simulink model "rtwdemo_autosar_client"  (Simulink 7.6)
settings: Solver=FixedStepDiscrete  SolverMode=SingleTasking  StartTime=0.0  StopTime=10.0  FixedStep=0.1  RelTol=1e-3
libraries: rtwdemo_autosar_csinterface x2, rtwlib x1
Description:
  | File Packaging for Models (Code and Data)
settings Model: Creator=The MathWorks Inc.  ExtModeAutoUpdateStatusClock=off
settings MATStruct: SampleTime=0.1  Offset=0  Priority=[20.0]
settings DataIOCC: LimitDataPoints=off  SaveFormat=StructureWithTime  SaveOutput=off  SaveTime=off  SignalLoggingName=logsOut
settings OptimizationCC: InlineParams=on  InlineInvariantSignals=on  StateBitsets=on  DataBitsets=on  UseTempVars=on  ZeroExternalMemoryAtStartup=off  ZeroInternalMemoryAtStartup=off  EfficientFloat2IntCast=on  EfficientMapNaN2IntZero=off  OptimizeModelRefInitCode=on  LifeSpan=floor((10.0)/86400)+1
settings DebuggingCC: CheckExecutionContextPreStartOutputMsg=on  CheckExecutionContextRuntimeOutputMsg=on  SolverPrmCheckMsg=none  StrictBusMsg=ErrorOnBusTreatedAsVector
settings HardwareCC: ProdIntDivRoundTo=Zero  ProdEndianess=LittleEndian  ProdHWDeviceType=Generic->32-bit Embedded Processor  TargetHWDeviceType=Generic->32-bit Embedded Processor
settings ModelReferenceCC: UpdateModelReferenceTargets=IfOutOfDate  CheckModelReferenceTargetMessage=none
settings RTWCC: SystemTargetFile=autosar.tlc  TLCOptions=-p0 -aWarnNonSaturatedBlocks=0  GenCodeOnly=on  TemplateMakefile=ert_default_tmf  Description=AUTOSAR  GenerateReport=on  RTWVerbose=off  ProcessScript=autosar_make_rtw_hook  IncludeHyperlinkInReport=on  LaunchReport=on  GenerateCodeInfo=on
settings CodeAppCC: ForceParamTrailComments=on  IgnoreCustomStorageClasses=off  MaxIdLength=128
settings STFCustomTargetCC: ParMdlRefBuildCompliant=on  CompOptLevelCompliant=on  IncludeMdlTerminateFcn=off  CombineOutputUpdateFcns=on  SuppressErrorStatus=on  ERTFirstTimeCompliant=on  ERTCustomFileBanners=on  SupportNonFinite=off  SupportComplex=off  SupportContinuousTime=off  SupportNonInlinedSFcns=off  AutosarCompliant=on  SystemTargetFile=autosar.tlc
settings ERTTargetCC: MultiwordLength=2048  IncludeMdlTerminateFcn=off  SuppressErrorStatus=on  SupportNonFinite=off  SupportComplex=off  ModelStepFunctionPrototypeControlCompliant=off  CPPClassGenCompliant=off  AutosarCompliant=on  ExtModeMexFile=noextcomm  InlinedParameterPlacement=NonHierarchical  ERTCustomFileTemplate=example_file_process.tlc  ERTFilePackagingFormat=CompactWithDataFile  ConvertIfToSwitch=off
settings CustomProperty: DataType=RTWOptions_EnumType__toolbox_rtw_targets_AUTOSAR_AUTOSAR_autosar_1_1AutosarSchemaVersion  Value=3.1
settings EnumStrPairs: String=2.0

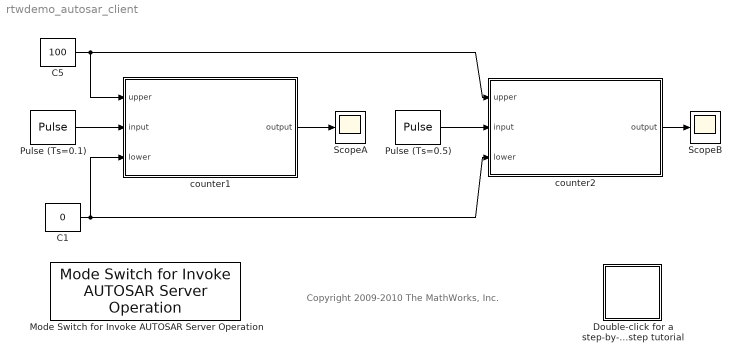
== system rtwdemo_autosar_client ==
  note: Copyright 2009-2010 The MathWorks, Inc.
  C1 : Constant  Value=0
  C5 : Constant  Value=100
  Double-click for a step-by-step tutorial : Subsystem
      settings: OpenFcn=showdemo('rtwdemo_autosar_clientserver_script');
      mask Type: Info
      mask Display: image(imread('targets_demo_info.bmp','bmp'),'center')
  Mode Switch for Invoke AUTOSAR Server Operation : rtwlib/AUTOSAR/Mode Switch for Invoke AUTOSAR Server Operation  SystemSampleTime=-1  mode=code generation  ShowInLibBrowser=on
  Pulse (Ts=0.1) : DiscretePulseGenerator  SampleTime=0.1  VectorParams1D=off
  Pulse (Ts=0.5) : DiscretePulseGenerator  SampleTime=0.5
  ScopeA : Scope
      settings: TimeRange=10  YMin=0  YMax=100
  ScopeB : Scope
      settings: TimeRange=10  YMin=0  YMax=25
  counter1 : Subsystem  Tag=AUTOSARConfigSubsystem  BlockChoice=|
      | rtwdemo_autosar_server_operation
      | (code generation)
      link override rtwdemo_autosar_server_operation (code generation): portName=Port1
      settings: AttributesFormatString=%<BlockChoice>  TemplateBlock=rtwdemo_autosar_csinterface/rtwdemo_autosar_server_operation
      settings: MemberBlocks=|
      | rtwdemo_autosar_server_operation
      | (code generation),rtwdemo_autosar_server_operation
      | (simulation)
  counter2 : Subsystem  Tag=AUTOSARConfigSubsystem  BlockChoice=|
      | rtwdemo_autosar_server_operation
      | (code generation)
      link override rtwdemo_autosar_server_operation (code generation): portName=Port2
      settings: AttributesFormatString=%<BlockChoice>  TemplateBlock=rtwdemo_autosar_csinterface/rtwdemo_autosar_server_operation
      settings: MemberBlocks=|
      | rtwdemo_autosar_server_operation
      | (code generation),rtwdemo_autosar_server_operation
      | (simulation)
  wires:
  counter1/1(output) -> ScopeA/1
  C1/1 -> counter1/3(lower), counter2/3(lower)
  C5/1 -> counter1/1(upper), counter2/1(upper)
  Pulse (Ts=0.1)/1 -> counter1/2(input)
  Pulse (Ts=0.5)/1 -> counter2/2(input)
  counter2/1(output) -> ScopeB/1

== system rtwdemo_autosar_client/Double-click for a step-by-step tutorial ==

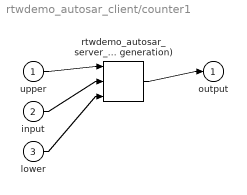
== system rtwdemo_autosar_client/counter1 ==
  upper : Inport
  input : Inport  Port=2
  lower : Inport  Port=3
  rtwdemo_autosar_server_operation (code generation) : rtwdemo_autosar_csinterface/rtwdemo_autosar_server_operation (code generation)  SystemSampleTime=-1  portName=Port1  operationPrototype=rtwdemo_autosar_server_operation(IN double upper, IN double input, IN double lower, OUT double output)  interfacePath=/rtwdemo_autosar/csinterface  serverType=Application software  showErrorStatus=off  SAMPLETIME=-1  showARPortLabels=off
  output : Outport
  wires:
  upper/1 -> rtwdemo_autosar_server_operation (code generation)/1
  input/1 -> rtwdemo_autosar_server_operation (code generation)/2
  lower/1 -> rtwdemo_autosar_server_operation (code generation)/3
  rtwdemo_autosar_server_operation (code generation)/1 -> output/1

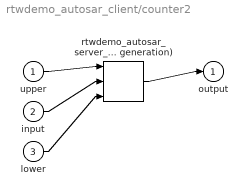
== system rtwdemo_autosar_client/counter2 ==
  upper : Inport
  input : Inport  Port=2
  lower : Inport  Port=3
  rtwdemo_autosar_server_operation (code generation) : rtwdemo_autosar_csinterface/rtwdemo_autosar_server_operation (code generation)  SystemSampleTime=-1  portName=Port2  operationPrototype=rtwdemo_autosar_server_operation(IN double upper, IN double input, IN double lower, OUT double output)  interfacePath=/rtwdemo_autosar/csinterface  serverType=Application software  showErrorStatus=off  SAMPLETIME=-1  showARPortLabels=off
  output : Outport
  wires:
  upper/1 -> rtwdemo_autosar_server_operation (code generation)/1
  input/1 -> rtwdemo_autosar_server_operation (code generation)/2
  lower/1 -> rtwdemo_autosar_server_operation (code generation)/3
  rtwdemo_autosar_server_operation (code generation)/1 -> output/1
